simulink model "gm_Config_Client"  (R2015b)
settings: Solver=VariableStepAuto  StartTime=0.0  StopTime=10.0  RelTol=1e-3
settings Model: Creator=Administrator  LastModifiedBy=Administrator
settings OptimizationCC: BlockReduction=off  ConditionallyExecuteInputs=off
settings DebuggingCC: InheritedTsInSrcMsg=none

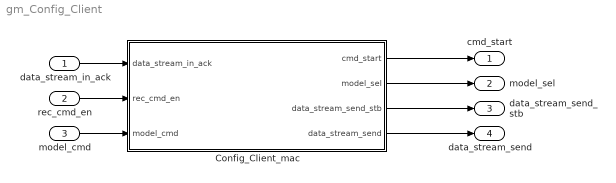
== system gm_Config_Client ==
  data_stream_in_ack : Inport  SampleTime=0
  rec_cmd_en : Inport  Port=2  SampleTime=0
  model_cmd : Inport  Port=3  SampleTime=0
  Config_Client_mac : Subsystem
  cmd_start : Outport
  model_sel : Outport  Port=2
  data_stream_send_stb : Outport  Port=3
  data_stream_send : Outport  Port=4
  wires:
  data_stream_in_ack/1 -> Config_Client_mac/1(data_stream_in_ack)
  rec_cmd_en/1 -> Config_Client_mac/2(rec_cmd_en)
  model_cmd/1 -> Config_Client_mac/3(model_cmd)
  Config_Client_mac/1(cmd_start) -> cmd_start/1
  Config_Client_mac/2(model_sel) -> model_sel/1
  Config_Client_mac/3(data_stream_send_stb) -> data_stream_send_stb/1
  Config_Client_mac/4(data_stream_send) -> data_stream_send/1

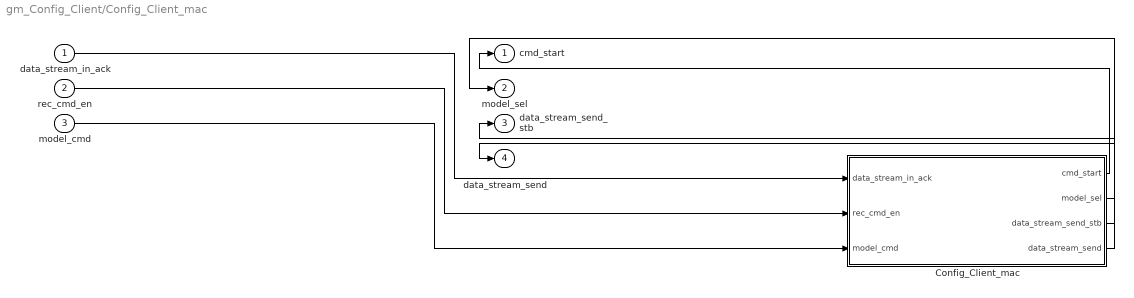
== system gm_Config_Client/Config_Client_mac ==
  data_stream_in_ack : Inport  SampleTime=0
  rec_cmd_en : Inport  Port=2  SampleTime=0
  model_cmd : Inport  Port=3  SampleTime=0
  Config_Client_mac : Stateflow chart  TreatAsAtomicUnit=on
  cmd_start : Outport
  model_sel : Outport  Port=2
  data_stream_send_stb : Outport  Port=3
  data_stream_send : Outport  Port=4
  wires:
  data_stream_in_ack/1 -> Config_Client_mac/1(data_stream_in_ack)
  rec_cmd_en/1 -> Config_Client_mac/2(rec_cmd_en)
  model_cmd/1 -> Config_Client_mac/3(model_cmd)
  Config_Client_mac/1(cmd_start) -> cmd_start/1
  Config_Client_mac/2(model_sel) -> model_sel/1
  Config_Client_mac/3(data_stream_send_stb) -> data_stream_send_stb/1
  Config_Client_mac/4(data_stream_send) -> data_stream_send/1

== stateflow chart gm_Config_Client/Config_Client_mac/Config_Client_mac ==
  settings: executeAtInitialization=1
  state Initial
    entry:
    data_stream_send_stb = 0;
    data_stream_send = uint8(0);
    cmd_start = 0;
    model_sel = 0;
    cnt_wait = uint32(0);
    cnt_halt = int32(0);
    %2.1.2
  state Tran_A
    entry:
    data_stream_send_stb = 1;
    data_stream_send = 65;%A
    cnt_wait = 0;
    cnt_halt = 0;
  state Tran_T
    entry:
    data_stream_send_stb = 1;
    data_stream_send = 84;%T
  state Tran_Enter
    entry: data_stream_send_stb = 1;
    data_stream_send = 13;%/r
  state Tran_Enter_1
    entry: data_stream_send_stb = 1;
    data_stream_send = 10;%/n
  state send_finish
    entry: data_stream_send_stb = 0;
    data_stream_send = 0;
  state wait_cnt1
    entry: cnt_wait = cnt_wait + 1;
    cnt_halt = 0;
    data_stream_send_stb = 0;
    data_stream_send = 0;
  state device_OK
    entry: model_sel = model_sel + 1;
    cnt_wait = uint32(0);
    cmd_start = 1;
  state Tran1_A
    entry:
    data_stream_send_stb = 1;
    data_stream_send = 65;%A
    cnt_wait = 0;
    cnt_halt = 0;
  state Tran1_Equal
    entry:
    data_stream_send_stb = 1;
    data_stream_send = 61;%=
  state Tran1_3
    entry:
    data_stream_send_stb = 1;
    data_stream_send = 51;%3
  state Tran1_Plus
    entry:
    data_stream_send_stb = 1;
    data_stream_send = 43;%+
  state Tran1_C
    entry:
    data_stream_send_stb = 1;
    data_stream_send = 67;%C
  state Tran1_W
    entry:
    data_stream_send_stb = 1;
    data_stream_send = 87;%W
  state Tran1_M
    entry:
    data_stream_send_stb = 1;
    data_stream_send = 77;%M
  state Tran1_O
    entry:
    data_stream_send_stb = 1;
    data_stream_send = 79;%O
  state Tran1_D
    entry:
    data_stream_send_stb = 1;
    data_stream_send = 68;%D
  state Tran1_E
    entry:
    data_stream_send_stb = 1;
    data_stream_send = 69;%E
  state Tran1_Enter
    entry: data_stream_send_stb = 1;
    data_stream_send = 13;%/r
  state Tran1_T
    entry:
    data_stream_send_stb = 1;
    data_stream_send = 84;%T
  state Tran1_Enter_1
    entry: data_stream_send_stb = 1;
    data_stream_send = 10;%/n
  state send_finish1
    entry: data_stream_send_stb = 0;
    data_stream_send = 0;
  state wait_cnt2
    entry: cnt_wait = cnt_wait + 1;
    cnt_halt = 0;
    data_stream_send_stb = 0;
    data_stream_send = 0;
  state device_OK1
    entry: model_sel = model_sel + 1;
    cnt_wait = uint32(0);
    cmd_start = 1;
  state Tran2_A
    entry:
    data_stream_send_stb = 1;
    data_stream_send = 65;%A
    cnt_wait = 0;
    cnt_halt = 0;
  state Tran2_C
    entry:
    data_stream_send_stb = 1;
    data_stream_send = 67;%C
  state Tran2_W
    entry:
    data_stream_send_stb = 1;
    data_stream_send = 87;%W
  state Tran2_T
    entry:
    data_stream_send_stb = 1;
    data_stream_send = 84;%T
  state Tran2_Plus
    entry:
    data_stream_send_stb = 1;
    data_stream_send = 43;%+
  state Tran2_J
    entry:
    data_stream_send_stb = 1;
    data_stream_send = 74;%J
  state Tran2_A1
    entry:
    data_stream_send_stb = 1;
    data_stream_send = 65;%A
  state Tran2_Equal
    entry:
    data_stream_send_stb = 1;
    data_stream_send = 61;%=
  state Tran2_Quota
    entry:
    data_stream_send_stb = 1;
    data_stream_send = 34;%"
  state Tran2_P
    entry:
    data_stream_send_stb = 1;
    data_stream_send = 80;%P
  state Tran2_U
    entry:
    data_stream_send_stb = 1;
    data_stream_send = 85;%U
  state Tran2_N
    entry:
    data_stream_send_stb = 1;
    data_stream_send = 78;%N
  state Tran2_Underline
    entry:
    data_stream_send_stb = 1;
    data_stream_send = 95;%_
  state Tran2_T1
    entry:
    data_stream_send_stb = 1;
    data_stream_send = 84;%T
  state Tran2_D
    entry:
    data_stream_send_stb = 1;
    data_stream_send = 68;%D
  state send_finish2
    entry: data_stream_send_stb = 0;
    data_stream_send = 0;
  state Tran2_O
    entry:
    data_stream_send_stb = 1;
    data_stream_send = 79;%O
  state Tran2_R
    entry:
    data_stream_send_stb = 1;
    data_stream_send = 82;%R
  state Tran2_Enter
    entry: data_stream_send_stb = 1;
    data_stream_send = 13;%/r
  state Tran2_Quota2
    entry:
    data_stream_send_stb = 1;
    data_stream_send = 34;%"
  state Tran2_Comma
    entry:
    data_stream_send_stb = 1;
    data_stream_send = 44;%,
  state Tran2_Quota1
    entry:
    data_stream_send_stb = 1;
    data_stream_send = 34;%"
  state Tran2_E
    entry:
    data_stream_send_stb = 1;
    data_stream_send = 69;%E
  state Tran2_N1
    entry:
    data_stream_send_stb = 1;
    data_stream_send = 78;%N
  state Tran2_Enter_1
    entry: data_stream_send_stb = 1;
    data_stream_send = 10;%/n
  state Tran2_Quota3
    entry:
    data_stream_send_stb = 1;
    data_stream_send = 34;%"
  state wait_cnt3
    entry: cnt_wait = cnt_wait + 1;
    cnt_halt = 0;
    data_stream_send_stb = 0;
    data_stream_send = 0;
  state device_OK2
    entry: model_sel = model_sel + 1;
    cnt_wait = uint32(0);
    cmd_start = 1;
  (default) -> Initial
  (junction 45) -> Initial
  Initial -> Tran_A
  Tran_T -> (junction 11)
  (junction 11) -> Tran_Enter [order 1] : [data_stream_in_ack == 1]
  Tran_A -> (junction 6)
  (junction 6) -> Tran_T [order 1] : [data_stream_in_ack == 1]
  Tran_Enter -> (junction 16)
  (junction 16) -> Tran_Enter_1 [order 1] : [data_stream_in_ack == 1]
  (junction 11) -> Tran_T [order 2] : [data_stream_in_ack == 0]
  (junction 6) -> Tran_A [order 2] : [data_stream_in_ack == 0]
  (junction 16) -> Tran_Enter [order 2] : [data_stream_in_ack == 0]
  (junction 21) -> Tran_Enter_1 [order 2] : [data_stream_in_ack == 0]
  Tran_Enter_1 -> (junction 21)
  (junction 27) -> Tran_A [order 1] : [model_cmd ~= 1] % ERROR or FAIL
  (junction 25) -> (junction 27) [order 1] : [rec_cmd_en == 1]
  send_finish -> (junction 25)
  (junction 21) -> send_finish [order 1] : [data_stream_in_ack == 1]
  (junction 25) -> send_finish [order 2] : [rec_cmd_en == 0]
  (junction 27) -> wait_cnt1 [order 2] : [model_cmd == 1] % receive OK
  (junction 34) -> wait_cnt1 [order 1] : [cnt_wait < 50000000]%0.05s
  wait_cnt1 -> (junction 34)
  (junction 34) -> (junction 39) [order 2] : [cnt_wait >=50000000]%0.05s
  (junction 39) -> device_OK
  device_OK -> Tran1_A
  Tran1_Equal -> (junction 164)
  (junction 164) -> Tran1_3 [order 1] : [data_stream_in_ack == 1]
  Tran1_T -> (junction 95)
  (junction 95) -> Tran1_Plus [order 1] : [data_stream_in_ack == 1]
  Tran1_Plus -> (junction 124)
  (junction 124) -> Tran1_C [order 1] : [data_stream_in_ack == 1]
  Tran1_C -> (junction 129)
  (junction 129) -> Tran1_W [order 1] : [data_stream_in_ack == 1]
  Tran1_O -> (junction 144)
  (junction 144) -> Tran1_D [order 1] : [data_stream_in_ack == 1]
  Tran1_D -> (junction 149)
  (junction 149) -> Tran1_E [order 1] : [data_stream_in_ack == 1]
  Tran1_E -> (junction 154)
  (junction 154) -> Tran1_Equal [order 1] : [data_stream_in_ack == 1]
  Tran1_M -> (junction 139)
  (junction 139) -> Tran1_O [order 1] : [data_stream_in_ack == 1]
  Tran1_W -> (junction 134)
  (junction 134) -> Tran1_M [order 1] : [data_stream_in_ack == 1]
  Tran1_3 -> (junction 169)
  (junction 169) -> Tran1_Enter [order 1] : [data_stream_in_ack == 1]
  (junction 164) -> Tran1_Equal [order 2] : [data_stream_in_ack == 0]
  Tran1_A -> (junction 97)
  (junction 97) -> Tran1_T [order 1] : [data_stream_in_ack == 1]
  (junction 95) -> Tran1_T [order 2] : [data_stream_in_ack == 0]
  (junction 124) -> Tran1_Plus [order 2] : [data_stream_in_ack == 0]
  (junction 129) -> Tran1_C [order 2] : [data_stream_in_ack == 0]
  (junction 149) -> Tran1_D [order 2] : [data_stream_in_ack == 0]
  (junction 154) -> Tran1_E [order 2] : [data_stream_in_ack == 0]
  Tran1_Enter -> (junction 98)
  (junction 98) -> Tran1_Enter_1 [order 1] : [data_stream_in_ack == 1]
  (junction 139) -> Tran1_M [order 2] : [data_stream_in_ack == 0]
  (junction 134) -> Tran1_W [order 2] : [data_stream_in_ack == 0]
  (junction 169) -> Tran1_3 [order 2] : [data_stream_in_ack == 0]
  (junction 97) -> Tran1_A [order 2] : [data_stream_in_ack == 0]
  (junction 144) -> Tran1_O [order 2] : [data_stream_in_ack == 0]
  (junction 98) -> Tran1_Enter [order 2] : [data_stream_in_ack == 0]
  (junction 96) -> Tran1_Enter_1 [order 1] : [data_stream_in_ack == 0]
  Tran1_Enter_1 -> (junction 96)
  (junction 99) -> Tran1_A [order 1] : [model_cmd ~= 1] % ERROR or FAIL
  (junction 100) -> (junction 99) [order 1] : [rec_cmd_en == 1]
  (junction 99) -> wait_cnt2 [order 2] : [model_cmd == 1] % receive OK
  (junction 96) -> send_finish1 [order 2] : [data_stream_in_ack == 1]
  send_finish1 -> (junction 100)
  (junction 100) -> send_finish1 [order 2] : [rec_cmd_en == 0]
  (junction 172) -> wait_cnt2 [order 1] : [cnt_wait < 50000000]%0.05s
  wait_cnt2 -> (junction 172)
  (junction 172) -> device_OK1 [order 2] : [cnt_wait >=50000000]%0.05s
  device_OK1 -> Tran2_A
  Tran2_C -> (junction 214)
  (junction 214) -> Tran2_W [order 2] : [data_stream_in_ack == 1]
  Tran2_A -> (junction 190)
  (junction 190) -> Tran2_T [order 1] : [data_stream_in_ack == 1]
  Tran2_Plus -> (junction 209)
  (junction 209) -> Tran2_C [order 2] : [data_stream_in_ack == 1]
  Tran2_T -> (junction 201)
  (junction 201) -> Tran2_Plus [order 1] : [data_stream_in_ack == 1]
  Tran2_W -> (junction 217)
  (junction 217) -> Tran2_J [order 1] : [data_stream_in_ack == 1]
  (junction 190) -> Tran2_A [order 2] : [data_stream_in_ack == 0]
  (junction 214) -> Tran2_C [order 1] : [data_stream_in_ack == 0]
  (junction 201) -> Tran2_T [order 2] : [data_stream_in_ack == 0]
  Tran2_J -> (junction 222)
  (junction 222) -> Tran2_A1 [order 1] : [data_stream_in_ack == 1]
  (junction 217) -> Tran2_W [order 2] : [data_stream_in_ack == 0]
  (junction 209) -> Tran2_Plus [order 1] : [data_stream_in_ack == 0]
  (junction 222) -> Tran2_J [order 2] : [data_stream_in_ack == 0]
  Tran2_A1 -> (junction 227)
  (junction 227) -> Tran2_P [order 1] : [data_stream_in_ack == 1]
  Tran2_P -> (junction 232)
  (junction 232) -> Tran2_Equal [order 1] : [data_stream_in_ack == 1]
  Tran2_Equal -> (junction 237)
  (junction 237) -> Tran2_Quota [order 1] : [data_stream_in_ack == 1]
  (junction 227) -> Tran2_A1 [order 2] : [data_stream_in_ack == 0]
  (junction 232) -> Tran2_P [order 2] : [data_stream_in_ack == 0]
  (junction 237) -> Tran2_Equal [order 2] : [data_stream_in_ack == 0]
  Tran2_Quota -> (junction 242)
  (junction 242) -> Tran2_U [order 1] : [data_stream_in_ack == 1]
  Tran2_U -> (junction 247)
  (junction 247) -> Tran2_N [order 1] : [data_stream_in_ack == 1]
  Tran2_N -> (junction 255)
  (junction 242) -> Tran2_Quota [order 2] : [data_stream_in_ack == 0]
  (junction 247) -> Tran2_U [order 2] : [data_stream_in_ack == 0]
  (junction 255) -> Tran2_N [order 1] : [data_stream_in_ack == 0]
  (junction 255) -> Tran2_T1 [order 2] : [data_stream_in_ack == 1]
  (junction 313) -> Tran2_A [order 1] : [model_cmd ~= 1] % ERROR or FAIL
  (junction 332) -> Tran2_Enter_1 [order 1] : [data_stream_in_ack == 0]
  (junction 256) -> Tran2_Underline [order 2] : [data_stream_in_ack == 1]
  Tran2_T1 -> (junction 256)
  (junction 256) -> Tran2_T1 [order 1] : [data_stream_in_ack == 0]
  (junction 259) -> Tran2_D [order 2] : [data_stream_in_ack == 1]
  Tran2_Underline -> (junction 259)
  (junction 331) -> Tran2_Enter [order 2] : [data_stream_in_ack == 0]
  (junction 259) -> Tran2_Underline [order 1] : [data_stream_in_ack == 0]
  (junction 264) -> Tran2_R [order 2] : [data_stream_in_ack == 1]
  Tran2_D -> (junction 264)
  (junction 264) -> Tran2_D [order 1] : [data_stream_in_ack == 0]
  (junction 266) -> Tran2_O [order 2] : [data_stream_in_ack == 1]
  Tran2_R -> (junction 266)
  (junction 274) -> Tran2_N1 [order 2] : [data_stream_in_ack == 1]
  Tran2_O -> (junction 274)
  (junction 309) -> (junction 313) [order 2] : [rec_cmd_en == 1]
  send_finish2 -> (junction 309)
  Tran2_Enter_1 -> (junction 332)
  (junction 266) -> Tran2_R [order 1] : [data_stream_in_ack == 0]
  (junction 332) -> send_finish2 [order 2] : [data_stream_in_ack == 1]
  (junction 274) -> Tran2_O [order 1] : [data_stream_in_ack == 0]
  (junction 309) -> send_finish2 [order 1] : [rec_cmd_en == 0]
  (junction 299) -> Tran2_Quota3 [order 2] : [data_stream_in_ack == 1]
  Tran2_Quota2 -> (junction 299)
  (junction 294) -> Tran2_Quota2 [order 2] : [data_stream_in_ack == 1]
  Tran2_Comma -> (junction 294)
  (junction 289) -> Tran2_Comma [order 2] : [data_stream_in_ack == 1]
  Tran2_Quota1 -> (junction 289)
  (junction 284) -> Tran2_Quota1 [order 2] : [data_stream_in_ack == 1]
  Tran2_E -> (junction 284)
  (junction 279) -> Tran2_E [order 2] : [data_stream_in_ack == 1]
  Tran2_N1 -> (junction 279)
  (junction 304) -> Tran2_Enter [order 1] : [data_stream_in_ack == 1]
  Tran2_Quota3 -> (junction 304)
  (junction 313) -> wait_cnt3 [order 2] : [model_cmd == 1] % receive OK
  (junction 299) -> Tran2_Quota2 [order 1] : [data_stream_in_ack == 0]
  (junction 294) -> Tran2_Comma [order 1] : [data_stream_in_ack == 0]
  (junction 289) -> Tran2_Quota1 [order 1] : [data_stream_in_ack == 0]
  (junction 284) -> Tran2_E [order 1] : [data_stream_in_ack == 0]
  (junction 279) -> Tran2_N1 [order 1] : [data_stream_in_ack == 0]
  (junction 304) -> Tran2_Quota3 [order 2] : [data_stream_in_ack == 0]
  (junction 331) -> Tran2_Enter_1 [order 1] : [data_stream_in_ack == 1]
  Tran2_Enter -> (junction 331)
  (junction 322) -> wait_cnt3 [order 1] : [cnt_wait < 50000000]%0.05s
  wait_cnt3 -> (junction 322)
  (junction 322) -> device_OK2 [order 2] : [cnt_wait >=50000000]%0.05s
  device_OK2 -> (junction 45)
  data: data_stream_in_ack input boolean; rec_cmd_en input boolean; model_cmd input fixdt(0,4,0); cmd_start output boolean; model_sel output fixdt(0,4,0); data_stream_send_stb output boolean; data_stream_send output uint8; cnt_wait local uint32; cnt_halt local int32
